simulink model "chap7_4sim"  (Simulink 7.0)
settings: Solver=ode45  StartTime=0.0  StopTime=10.0  RelTol=1e-3
libraries: simulink x1
settings Model: Creator=hp  LastModifiedBy=eleliuj
settings DataIOCC: SignalLoggingName=sigsOut
settings DebuggingCC: SaveWithParameterizedLinksMsg=none  SignalResolutionControl=TryResolveAllWithWarning  SolverPrmCheckMsg=none  MultiTaskDSMMsg=warning  MultiTaskCondExecSysMsg=none  StrictBusMsg=None
settings HardwareCC: TargetUnknown=on
settings RTWCC: IncludeERTFirstTime=on
settings GRTTargetCC: TargetFcnLib=ansi_tfl_tmw.mat

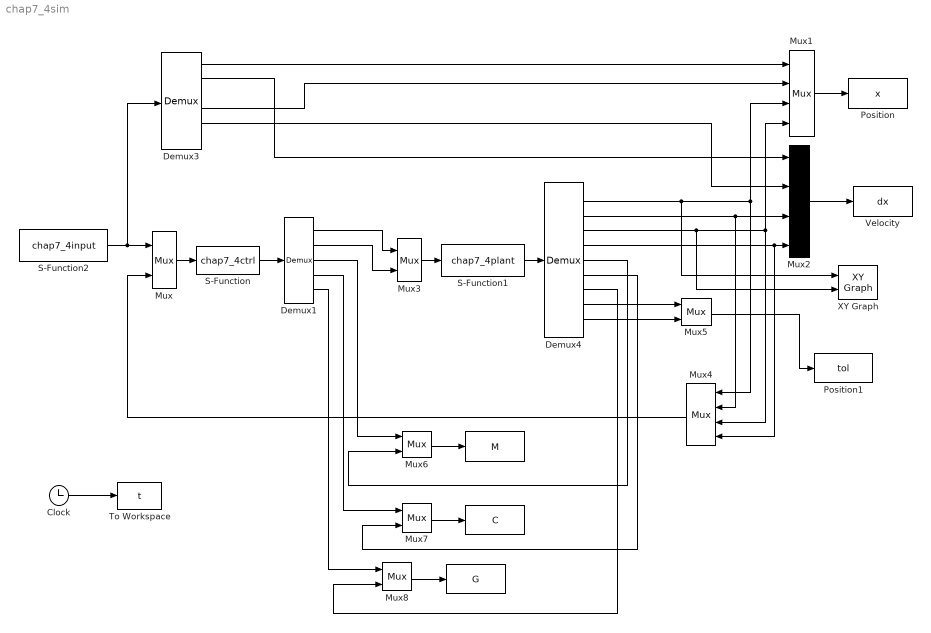
== system chap7_4sim ==
  " " : ToWorkspace  VariableName=M  SampleTime=-1  SaveFormat=Array
  "  " : ToWorkspace  VariableName=C  SampleTime=-1  SaveFormat=Array
  "   " : ToWorkspace  VariableName=G  SampleTime=-1  SaveFormat=Array
  Clock : Clock
      settings: Decimation=10
  Demux1 : Demux  Outputs=5
  Demux3 : Demux  Outputs=6
  Demux4 : Demux  Outputs=9
  Mux{,3,5..8} (6 alike) : Mux  Inputs=2
  Mux1 : Mux
  Mux2 : Mux
  Mux4 : Mux  Orientation=left
  Position : ToWorkspace  VariableName=x  SampleTime=-1  SaveFormat=Array
  Position1 : ToWorkspace  VariableName=tol  SampleTime=-1  SaveFormat=Array
  S-Function : S-Function  FunctionName=chap7_4ctrl
  S-Function1 : S-Function  FunctionName=chap7_4plant
  S-Function2 : S-Function  FunctionName=chap7_4input
  To Workspace : ToWorkspace  VariableName=t  SampleTime=-1  SaveFormat=Array
  Velocity : ToWorkspace  VariableName=dx  SampleTime=-1  SaveFormat=Array
  XY Graph : simulink/Sinks/XY Graph  SystemSampleTime=-1  xmin=0.75  xmax=1.25  ymin=0.75  ymax=1.25  st=-1
  wires:
  S-Function2/1 -> Demux3/1, Mux/1
  Mux/1 -> S-Function/1
  Demux3/1 -> Mux1/1
  Demux3/4 -> Mux1/2
  Demux4/1 -> Mux4/1, Mux1/3, XY Graph/1
  Demux4/3 -> Mux4/3, Mux1/4, XY Graph/2
  Demux3/2 -> Mux2/1
  Demux3/5 -> Mux2/2
  Mux2/1 -> Velocity/1
  Demux4/2 -> Mux2/3, Mux4/2
  Demux4/4 -> Mux2/4, Mux4/4
  S-Function/1 -> Demux1/1
  Demux1/1 -> Mux3/1
  Mux3/1 -> S-Function1/1
  S-Function1/1 -> Demux4/1
  Mux4/1 -> Mux/2
  Mux6/1 -> " "/1
  Demux1/3 -> Mux6/1
  Demux4/5 -> Mux6/2
  Mux7/1 -> "  "/1
  Demux1/4 -> Mux7/1
  Mux8/1 -> "   "/1
  Demux1/5 -> Mux8/1
  Mux1/1 -> Position/1
  Demux4/6 -> Mux7/2
  Demux4/7 -> Mux8/2
  Clock/1 -> To Workspace/1
  Mux5/1 -> Position1/1
  Demux1/2 -> Mux3/2
  Demux4/8 -> Mux5/1
  Demux4/9 -> Mux5/2
